simulink model "verify_WDB_Creator_mdl"  (R2016b)
settings: Solver=VariableStepDiscrete  StartTime=0.0  StopTime=1  MaxStep=1  RelTol=1e-3  EnableMultiTasking=on
libraries: carnot x1
settings Model: Creator=drhf  LastModifiedBy=srrt
settings DataIOCC: SaveFormat=Array  SignalLoggingSaveFormat=ModelDataLogs
settings OptimizationCC: ExpressionDepthLimit=2147483647  LifeSpan=inf
settings DebuggingCC: UnderspecifiedInitializationDetection=Classic  MergeDetectMultiDrivingBlocksExec=none  SolverPrmCheckMsg=warning  FcnCallInpInsideContextMsg=warning  StateNameClashWarn=warning  SFUnexpectedBacktrackingDiag=warning  SFNoUnconditionalDefaultTransitionDiag=warning  SFExecutionAtInitializationDiag=none
settings HardwareCC: ProdBitPerPointer=32  ProdBitPerSizeT=32  ProdBitPerPtrDiffT=32  ProdLargestAtomicFloat=None  ProdIntDivRoundTo=Undefined  ProdEndianess=Unspecified  ProdWordSize=32  ProdHWDeviceType=32-bit Generic
settings ModelReferenceCC: PropagateSignalLabelsOutOfModel=off
settings GRTTargetCC: TargetLangStandard=C89/C90 (ANSI)  GeneratePreprocessorConditionals=Disable all  CombineOutputUpdateFcns=off  GRTInterface=on
settings ConfigComp: CovMetricSettings=dw  CovHtmlReporting=on  CovSaveCumulativeToWorkspaceVar=on  CovSaveSingleToWorkspaceVar=on  CovExternalEMLEnable=off

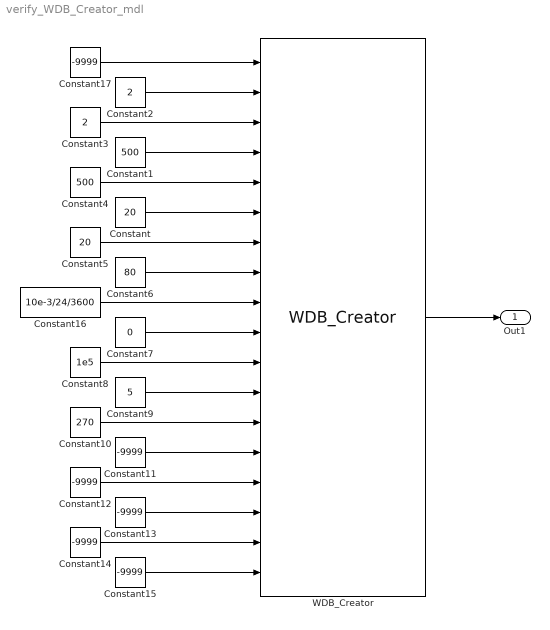
== system verify_WDB_Creator_mdl ==
  Constant : Constant  Value=20
  Constant1 : Constant  Value=500
  Constant10 : Constant  Value=270
  Constant{11..15,17} (6 alike) : Constant  Value=-9999
  Constant16 : Constant  Value=10e-3/24/3600
  Constant2 : Constant  Value=2
  Constant3 : Constant  Value=2
  Constant4 : Constant  Value=500
  Constant5 : Constant  Value=20
  Constant6 : Constant  Value=80
  Constant7 : Constant  Value=0
  Constant8 : Constant  Value=1e5
  Constant9 : Constant  Value=5
  WDB_Creator : carnot/Basic/Weather_and_Sun/WDB_Creator
  Out1 : Outport
  wires:
  WDB_Creator/1 -> Out1/1
  Constant2/1 -> WDB_Creator/2
  Constant3/1 -> WDB_Creator/3
  Constant1/1 -> WDB_Creator/4
  Constant4/1 -> WDB_Creator/5
  Constant/1 -> WDB_Creator/6
  Constant5/1 -> WDB_Creator/7
  Constant6/1 -> WDB_Creator/8
  Constant7/1 -> WDB_Creator/10
  Constant8/1 -> WDB_Creator/11
  Constant9/1 -> WDB_Creator/12
  Constant10/1 -> WDB_Creator/13
  Constant11/1 -> WDB_Creator/14
  Constant16/1 -> WDB_Creator/9
  Constant15/1 -> WDB_Creator/18
  Constant13/1 -> WDB_Creator/16
  Constant14/1 -> WDB_Creator/17
  Constant12/1 -> WDB_Creator/15
  Constant17/1 -> WDB_Creator/1
